simulink model "TF_Vs_SS"  (R2021a)
settings: Solver=VariableStepAuto  StartTime=0.0  StopTime=10.0  MaxStep=10e-3  RelTol=1e-3
settings Model: Creator=User  LastModifiedBy=User

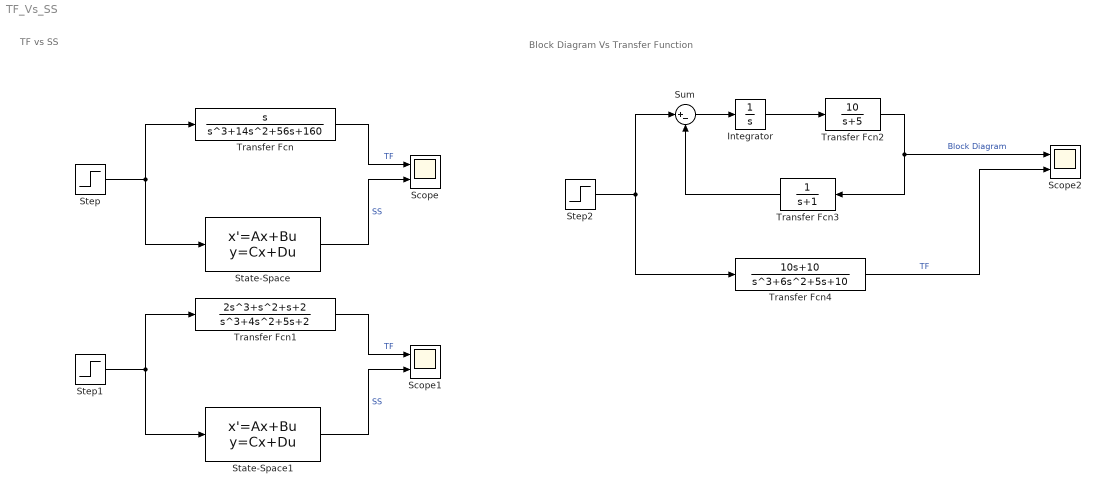
== system TF_Vs_SS ==
  note: Block Diagram Vs Transfer Function
  note: TF vs SS
  Integrator : Integrator
  Scope : Scope  NumInputPorts=2
  Scope1 : Scope  NumInputPorts=2
  Scope2 : Scope  NumInputPorts=2
  State-Space : StateSpace  A=[0 1 0;0 0 1;-160 -56 -14;]  B=[0; 1; -14]  C=[1 0 0]  D=[0]  InitialCondition=0  ParameterTunability=Optimized
  State-Space1 : StateSpace  A=[0 1 0;0 0 1;-2 -5 -4;]  B=[-7; 19; -43]  C=[1 0 0]  D=[2]  InitialCondition=0  ParameterTunability=Optimized
  Step : Step  SampleTime=0
  Step1 : Step  SampleTime=0
  Step2 : Step  SampleTime=0
  Sum : Sum  Inputs=|+-
  Transfer Fcn : TransferFcn  Numerator=[1 0]  Denominator=[1 14 56 160]
  Transfer Fcn1 : TransferFcn  Numerator=[2 1 1 2]  Denominator=[1 4 5 2]
  Transfer Fcn2 : TransferFcn  Numerator=[10]  Denominator=[1 5]
  Transfer Fcn3 : TransferFcn  Denominator=[1 1]
  Transfer Fcn4 : TransferFcn  Numerator=[10 10]  Denominator=[1 6 5 10]
  wires:
  Step/1 -> State-Space/1, Transfer Fcn/1
  State-Space/1 -> Scope/2  "SS"
  Transfer Fcn/1 -> Scope/1  "TF"
  Transfer Fcn1/1 -> Scope1/1  "TF"
  State-Space1/1 -> Scope1/2  "SS"
  Step1/1 -> Transfer Fcn1/1, State-Space1/1
  Integrator/1 -> Transfer Fcn2/1
  Sum/1 -> Integrator/1
  Transfer Fcn3/1 -> Sum/2
  Transfer Fcn2/1 -> Transfer Fcn3/1, Scope2/1  "Block Diagram"
  Transfer Fcn4/1 -> Scope2/2  "TF"
  Step2/1 -> Sum/1, Transfer Fcn4/1
